simulink model "Ralenti_BO_End"  (R2024b)
settings: Solver=FixedStepAuto  StartTime=0.0  StopTime=80  FixedStep=10e-3  RelTol=1e-5  AbsTol=1e-6
values from neighbouring files (symbols this model uses):
  Copti = [0.4 1.0 1.5 2.9 3.5 4.1 5.2 5.4 7.5  8.5  9.1  9.9 10.1 11.8 11.9 ... (first row only)    [InitISM_AII.m]
  gam = 1.4    [InitISM_AII.m]
  J = 0.18    [InitISM_AII.m]
  Kv = 0.0016    [InitISM_AII.m]
  MAPtc = 0.03    [InitISM_AII.m]
  Mim0 = 0+0.001    (= 0.001)    [InitISM_AII.m]
  nv_remp = [0.090 0.110 0.120 0.110 0.130 0.150 0.135 0.155 0.140 0.145 0.140 0.135 0.120 0.120 ... (first row only)    [InitISM_AII.m]
  Pamb = 101300    [InitISM_AII.m]
  Pim0 = 0.8e5    (= 80000)    [InitISM_AII.m]
  PRcrit = ((gam+1)/2)^(gam/(1-gam))    (= 0.528281787717)    [InitISM_AII.m]
  Psens0 = 1e5    (= 100000)    [InitISM_AII.m]
  Rair = 287.0    (= 287)    [InitISM_AII.m]
  table_rdt_AA = [1.0000 0.9980 0.9955 0.9680 0.9500 0.9020 0.8195 0.6875 0.6080 0.5195 0.2000 0.0755]    [InitISM_AII.m]
  Tamb = 300    [InitISM_AII.m]
  Vcol = 0.0035    [InitISM_AII.m]
  Vcyl = 1998e-6/4    (= 0.0004995)    [InitISM_AII.m]
  vect_delta_AA = [0 2 3 8 10 14 19 25 28 31 40 43]    [InitISM_AII.m]
undefined symbols (not defined in the file or in its folder): N0
settings Model: Creator=a030141  LastModifiedBy=ramse
settings SolverCC: AutoScaleAbsTol=off  AlgebraicLoopSolver=TrustRegion
settings DataIOCC: SaveFormat=Array  SignalLoggingSaveFormat=ModelDataLogs  ReturnWorkspaceOutputs=off  SignalLoggingName=sigsOut
settings OptimizationCC: BlockReduction=off  BooleanDataType=off  ReuseModelBlockBuffer=off  ExpressionDepthLimit=2147483647  InitFltsAndDblsToZero=on  LifeSpan=inf
settings DebuggingCC: SaveWithParameterizedLinksMsg=none  UnderspecifiedInitializationDetection=Classic  MergeDetectMultiDrivingBlocksExec=none  SignalResolutionControl=TryResolveAllWithWarning  MultiTaskDSMMsg=warning  MultiTaskCondExecSysMsg=none  FcnCallInpInsideContextMsg=warning  UnconnectedInputMsg=warning  UnconnectedOutputMsg=warning  UnconnectedLineMsg=warning  StateNameClashWarn=warning  SFUnexpectedBacktrackingDiag=warning  SFNoUnconditionalDefaultTransitionDiag=warning  SFExecutionAtInitializationDiag=none  ArithmeticOperatorsInVariantConditions=warning
settings HardwareCC: ProdBitPerPointer=32  ProdBitPerSizeT=32  ProdBitPerPtrDiffT=32  ProdLargestAtomicFloat=None  ProdIntDivRoundTo=Undefined  ProdEndianess=Unspecified  ProdWordSize=32  ProdHWDeviceType=32-bit Generic  TargetUnknown=on
settings ModelReferenceCC: EnableRefExpFcnMdlSchedulingChecks=on  PropagateSignalLabelsOutOfModel=off
settings SFSimCC: SimUseLocalCustomCode=off  CustomCodeUndefinedFunction=UseInterfaceOnly
settings RTWCC: TemplateMakefile=grt_vc.tmf  RTWUseLocalCustomCode=off  GPUComputeCapability=3.5  DLArmComputeVersion=19.05
settings CodeAppCC: StateflowObjectComments=on
settings GRTTargetCC: TargetFcnLib=ansi_tfl_tmw.mat  TargetLangStandard=C89/C90 (ANSI)  CombineOutputUpdateFcns=off  GRTInterface=on
settings ConfigComp: CovMetricSettings=dw  CovSaveCumulativeToWorkspaceVar=on  CovSaveSingleToWorkspaceVar=on  CovExternalEMLEnable=off

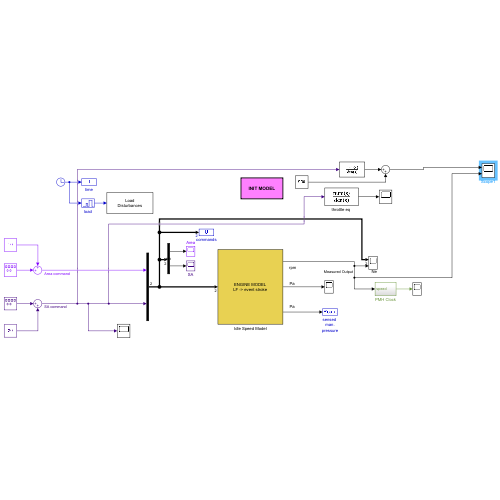
[thumbnail: Simulink's stored preview of the top-level diagram]
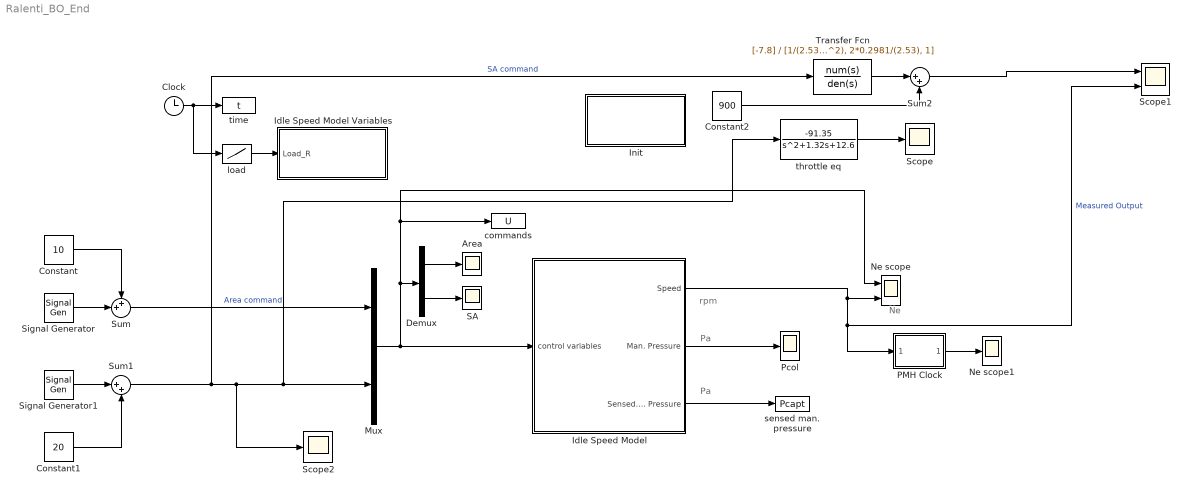
== system Ralenti_BO_End ==
  note: Pa
  note: Pa
  note: rpm
  note: Ne
  Area : Scope
  Clock : Clock
  Constant : Constant  Value=10  SampleTime=-1
  Constant1 : Constant  Value=20
  Constant2 : Constant  Value=900
  Demux : Demux  Outputs=2
      settings: DisplayOption=none
  Idle Speed Model : Subsystem
      mask Display: disp('ENGINE MODEL\nLF -> event stroke')
  Idle Speed Model Variables : Subsystem
      mask Display: disp('Load\nDisturbances')
  Init : Subsystem  TreatAsAtomicUnit=on
      settings: OpenFcn=InitISM_AII
      mask Display: disp('INIT MODEL')
  Mux : Mux  Inputs=2
  Ne scope : Scope  NumInputPorts=2
  Ne scope1 : Scope
  PMH Clock : Subsystem
  Pcol : Scope
  SA : Scope
  Scope : Scope
  Scope1 : Scope  NumInputPorts=2
  Scope2 : Scope
  Signal Generator : SignalGenerator  WaveForm=square  Amplitude=0  Frequency=0.01
  Signal Generator1 : SignalGenerator  WaveForm=square  Amplitude=2  Frequency=0.01
  Sum : Sum  Inputs=++|  SaturateOnIntegerOverflow=on
  Sum1 : Sum  Inputs=|++  SaturateOnIntegerOverflow=on
  Sum2 : Sum  Inputs=|++
  Transfer Fcn : TransferFcn  Numerator=[-7.8]  Denominator=[1/(2.53^2), 2*0.2981/(2.53), 1]
  commands : ToWorkspace  VariableName=U  SampleTime=-1
  load : Lookup  InputValues="[0  20 20 30 30 40 40 60 60 70]"  Table=[0 0 5 5 0 0 10 10 0 0]
  sensed man. pressure : ToWorkspace  VariableName=Pcapt  SampleTime=-1
  "throttle eq " : TransferFcn  Numerator=[-91.35]  Denominator=[1 1.32 12.6]
  time : ToWorkspace  VariableName=t  SampleTime=-1
  wires:
  Idle Speed Model/2(Man. Pressure) -> Pcol/1
  PMH Clock/1(out_1) -> Ne scope1/1
  Clock/1 -> time/1, load/1
  Idle Speed Model/3(Sensed Man. Pressure) -> sensed man. pressure/1
  Demux/1 -> Area/1
  Demux/2 -> SA/1
  load/1 -> Idle Speed Model Variables/1(Load_R)
  Mux/1 -> Idle Speed Model/1(control variables), Demux/1, Ne scope/1, commands/1
  Signal Generator1/1 -> Sum1/1
  Constant/1 -> Sum/1
  Constant1/1 -> Sum1/2
  Sum1/1 -> Transfer Fcn/1, Scope2/1, "throttle eq "/1, Mux/2  "SA command"
  Idle Speed Model/1(Speed) -> Ne scope/2, PMH Clock/1(speed), Scope1/2  "Measured Output"
  Sum/1 -> Mux/1  "Area command"
  Signal Generator/1 -> Sum/2
  "throttle eq "/1 -> Scope/1
  Transfer Fcn/1 -> Sum2/1
  Constant2/1 -> Sum2/2
  Sum2/1 -> Scope1/1

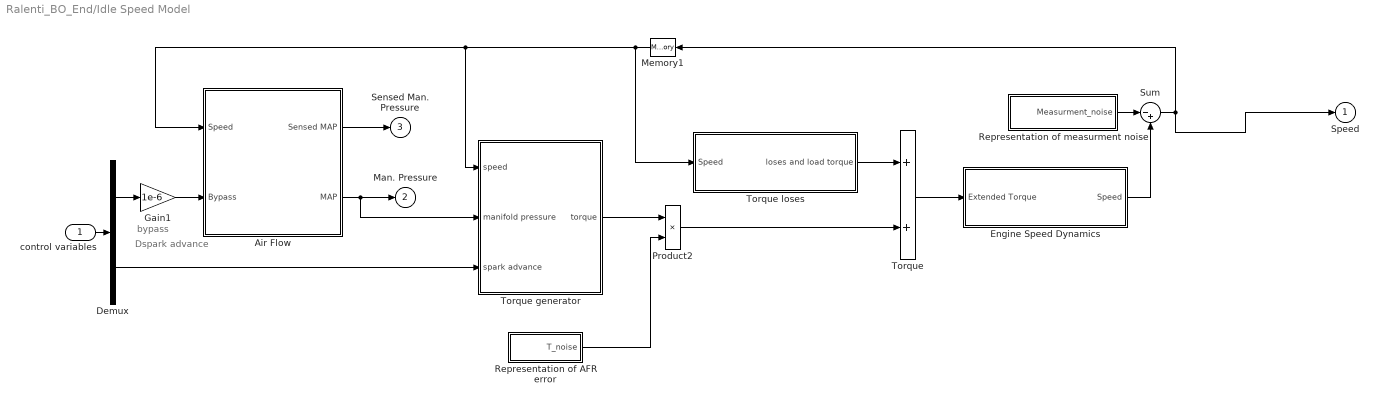
== system Ralenti_BO_End/Idle Speed Model ==
  note: Dspark advance
  note: bypass
  control variables : Inport
  " Torque loses" : Subsystem
  Air Flow : Subsystem
  Demux : Demux  Outputs=2
      settings: DisplayOption=none
  Engine Speed Dynamics : Subsystem
  Gain1 : Gain  Gain=1e-6  SaturateOnIntegerOverflow=on  OutDataTypeStr=Inherit: Same as input  ParamDataTypeStr=Inherit: Same as input
  Memory1 : Memory  InheritSampleTime=on
  Product2 : Product  Inputs=**  InputSameDT=on  SaturateOnIntegerOverflow=on  OutDataTypeStr=Inherit: Same as first input
  Representation of AFR error : Subsystem
  Representation of measurment noise : Subsystem
  Sum : Sum  Inputs=|-+  InputSameDT=on  SaturateOnIntegerOverflow=on  OutDataTypeStr=Inherit: Same as first input
  Torque : Sum  InputSameDT=on  SaturateOnIntegerOverflow=on  OutDataTypeStr=Inherit: Same as first input
  Torque generator : Subsystem
  Speed : Outport  VectorParamsAs1DForOutWhenUnconnected=off
  Man. Pressure : Outport  Port=2  VectorParamsAs1DForOutWhenUnconnected=off
  Sensed Man. Pressure : Outport  Port=3  VectorParamsAs1DForOutWhenUnconnected=off
  wires:
  Gain1/1 -> Air Flow/2(Bypass)
  Demux/1 -> Gain1/1
  Air Flow/2(MAP) -> Man. Pressure/1, Torque generator/2(manifold pressure)
  Air Flow/1(Sensed MAP) -> Sensed Man. Pressure/1
  Demux/2 -> Torque generator/3(spark advance)
  control variables/1 -> Demux/1
  Torque generator/1(torque) -> Product2/1
  Product2/1 -> Torque/2
  Representation of AFR error/1(T_noise) -> Product2/2
  Representation of measurment noise/1(Measurment_noise) -> Sum/1
  " Torque loses"/1(loses and load torque) -> Torque/1
  Torque/1 -> Engine Speed Dynamics/1(Extended Torque)
  Engine Speed Dynamics/1(Speed) -> Sum/2
  Memory1/1 -> Air Flow/1(Speed), Torque generator/1(speed), " Torque loses"/1(Speed)
  Sum/1 -> Speed/1, Memory1/1

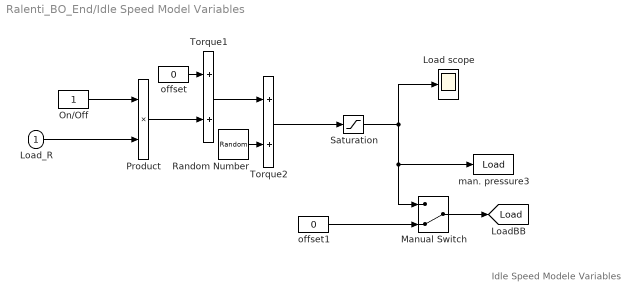
== system Ralenti_BO_End/Idle Speed Model Variables ==
  note: Idle Speed Modele Variables
  Load_R : Inport
  Load scope : Scope
  Manual Switch : ManualSwitch  CurrentSetting=0
  On/Off : Constant
  Product : Product  InputSameDT=on  SaturateOnIntegerOverflow=on  OutDataTypeStr=Inherit: Same as first input
  Random Number : RandomNumber  Variance=0.001  SampleTime=0.01
  Saturation : Saturate  UpperLimit=30  LowerLimit=0
  Torque1 : Sum  InputSameDT=on  SaturateOnIntegerOverflow=on  OutDataTypeStr=Inherit: Same as first input
  Torque2 : Sum  InputSameDT=on  SaturateOnIntegerOverflow=on  OutDataTypeStr=Inherit: Same as first input
  man. pressure3 : ToWorkspace  VariableName=Load  SampleTime=-1
  offset : Constant  Value=0
  offset1 : Constant  Value=0
  tag scope: Load=global
  wires:
  On/Off/1 -> Product/1
  Load_R/1 -> Product/2
  Product/1 -> Torque1/2
  offset/1 -> Torque1/1
  Random Number/1 -> Torque2/2
  Torque1/1 -> Torque2/1
  Saturation/1 -> Load scope/1, man. pressure3/1, Manual Switch/1
  Torque2/1 -> Saturation/1
  Manual Switch/1 -> [Load]
  offset1/1 -> Manual Switch/2

== system Ralenti_BO_End/Init ==

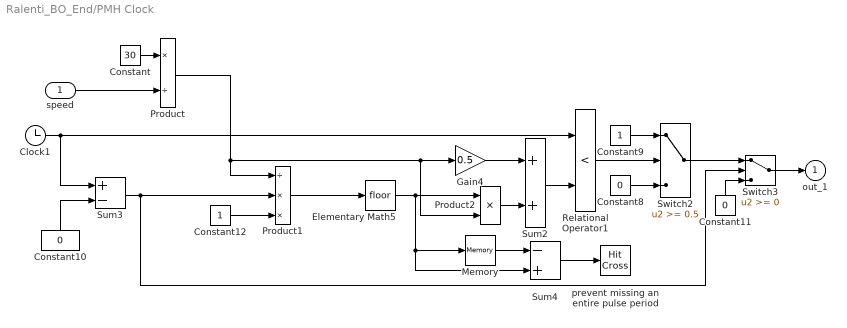
== system Ralenti_BO_End/PMH Clock ==
  speed : Inport
  Clock1 : Clock
  Constant : Constant  Value=30
  Constant10 : Constant  Value=0
  Constant11 : Constant  Value=0
  Constant12 : Constant
  Constant8 : Constant  Value=0
  Constant9 : Constant
  Elementary Math5 : Rounding
  Gain4 : Gain  Gain=0.5  SaturateOnIntegerOverflow=on  OutDataTypeStr=Inherit: Same as input  ParamDataTypeStr=Inherit: Same as input
  Memory : Memory
  Product : Product  Inputs=*/  InputSameDT=on  SaturateOnIntegerOverflow=on  OutDataTypeStr=Inherit: Same as first input
  Product1 : Product  Inputs=/**  InputSameDT=on  SaturateOnIntegerOverflow=on  OutDataTypeStr=Inherit: Same as first input
  Product2 : Product  InputSameDT=on  SaturateOnIntegerOverflow=on  OutDataTypeStr=Inherit: Same as first input
  Relational Operator1 : RelationalOperator  Operator=<
  Sum2 : Sum  InputSameDT=on  SaturateOnIntegerOverflow=on  OutDataTypeStr=Inherit: Same as first input
  Sum3 : Sum  Inputs=+-  InputSameDT=on  SaturateOnIntegerOverflow=on  OutDataTypeStr=Inherit: Same as first input
  Sum4 : Sum  Inputs=-+  InputSameDT=on  SaturateOnIntegerOverflow=on  OutDataTypeStr=Inherit: Same as first input
  Switch2 : Switch  Threshold=0.5
  Switch3 : Switch
  prevent missing an entire pulse period : HitCross  HitCrossingOffset=1  ShowOutputPort=off
  out_1 : Outport  VectorParamsAs1DForOutWhenUnconnected=off
  wires:
  Elementary Math5/1 -> Sum4/2, Memory/1, Product2/1
  Gain4/1 -> Sum2/1
  Product1/1 -> Elementary Math5/1
  Switch2/1 -> Switch3/1
  Constant11/1 -> Switch3/3
  Constant9/1 -> Switch2/1
  Constant8/1 -> Switch2/3
  Relational Operator1/1 -> Switch2/2
  Switch3/1 -> out_1/1
  Sum2/1 -> Relational Operator1/2
  Clock1/1 -> Relational Operator1/1, Sum3/1
  Sum3/1 -> Switch3/2, Product1/2
  Constant10/1 -> Sum3/2
  Memory/1 -> Sum4/1
  Sum4/1 -> prevent missing an entire pulse period/1
  Product2/1 -> Sum2/2
  Constant12/1 -> Product1/3
  Constant/1 -> Product/1
  speed/1 -> Product/2
  Product/1 -> Product1/1, Gain4/1, Product2/2

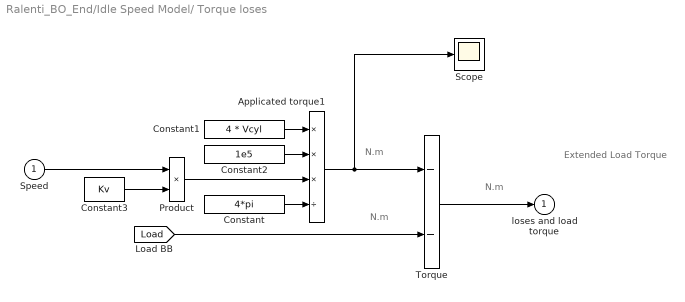
== system Ralenti_BO_End/Idle Speed Model/ Torque loses ==
  note: N.m
  note: Extended Load Torque
  note: N.m
  note: N.m
  Speed : Inport
  Applicated torque1 : Product  Inputs=***/  InputSameDT=on  SaturateOnIntegerOverflow=on  OutDataTypeStr=Inherit: Same as first input
  Constant : Constant  Value=4*pi
  Constant1 : Constant  Value=4 * Vcyl
  Constant2 : Constant  Value=1e5
  Constant3 : Constant  Value=Kv
  Product : Product  Inputs=**  InputSameDT=on  RndMeth=Zero  SaturateOnIntegerOverflow=on  OutDataTypeStr=Inherit: Same as first input
  Scope : Scope
  Torque : Sum  Inputs=--  InputSameDT=on  SaturateOnIntegerOverflow=on  OutDataTypeStr=Inherit: Same as first input
  loses and load torque : Outport  VectorParamsAs1DForOutWhenUnconnected=off
  wires:
  Constant3/1 -> Product/2
  Speed/1 -> Product/1
  [Load] -> Torque/2
  Torque/1 -> loses and load torque/1
  Product/1 -> Applicated torque1/3
  Applicated torque1/1 -> Torque/1, Scope/1
  Constant/1 -> Applicated torque1/4
  Constant1/1 -> Applicated torque1/1
  Constant2/1 -> Applicated torque1/2

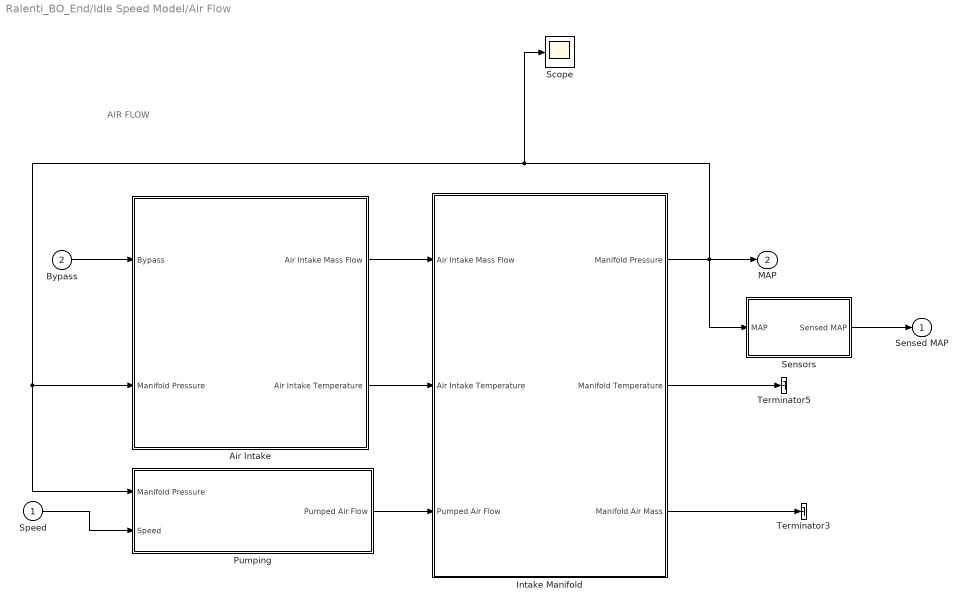
== system Ralenti_BO_End/Idle Speed Model/Air Flow ==
  note: AIR FLOW
  Speed : Inport
  Bypass : Inport  Port=2
  Air Intake : Subsystem
  Intake Manifold : Subsystem
  Pumping : Subsystem
  Scope : Scope
  Sensors : Subsystem
  Terminator3 : Terminator
  Terminator5 : Terminator
  Sensed MAP : Outport  VectorParamsAs1DForOutWhenUnconnected=off
  MAP : Outport  Port=2  VectorParamsAs1DForOutWhenUnconnected=off
  wires:
  Pumping/1(Pumped Air Flow) -> Intake Manifold/3(Pumped Air Flow)
  Sensors/1(Sensed MAP) -> Sensed MAP/1
  Air Intake/1(Air Intake Mass Flow) -> Intake Manifold/1(Air Intake Mass Flow)
  Bypass/1 -> Air Intake/1(Bypass)
  Air Intake/2(Air Intake Temperature) -> Intake Manifold/2(Air Intake Temperature)
  Intake Manifold/2(Manifold Temperature) -> Terminator5/1
  Intake Manifold/3(Manifold Air Mass) -> Terminator3/1
  Speed/1 -> Pumping/2(Speed)
  Intake Manifold/1(Manifold Pressure) -> MAP/1, Sensors/1(MAP), Scope/1, Pumping/1(Manifold Pressure), Air Intake/2(Manifold Pressure)

== system Ralenti_BO_End/Idle Speed Model/Engine Speed Dynamics ==
  note: Engine Speed
  note: Tr/min
  note: rad/s
  Extended Torque : Inport
  Constant : Constant  Value=J
  Product1 : Product  Inputs=*/  InputSameDT=on  SaturateOnIntegerOverflow=on  OutDataTypeStr=Inherit: Same as first input
  integrator : Integrator  InitialCondition=N0  UpperSaturationLimit=100  LowerSaturationLimit=0
  speed unit conversion : Gain  Gain=30/pi  SaturateOnIntegerOverflow=on  OutDataTypeStr=Inherit: Same as input  ParamDataTypeStr=Inherit: Same as input
  Speed : Outport  VectorParamsAs1DForOutWhenUnconnected=off
  wires:
  Constant/1 -> Product1/2
  Extended Torque/1 -> Product1/1
  Product1/1 -> speed unit conversion/1
  speed unit conversion/1 -> integrator/1
  integrator/1 -> Speed/1

== system Ralenti_BO_End/Idle Speed Model/Representation of AFR error ==
  Constant : Constant
  Random Number : RandomNumber  Variance=0  SampleTime=0.01
  Sum : Sum  Inputs=|-+  InputSameDT=on  SaturateOnIntegerOverflow=on  OutDataTypeStr=Inherit: Same as first input
  T_noise : Outport  VectorParamsAs1DForOutWhenUnconnected=off
  wires:
  Random Number/1 -> Sum/1
  Sum/1 -> T_noise/1
  Constant/1 -> Sum/2

== system Ralenti_BO_End/Idle Speed Model/Representation of measurment noise ==
  Random Number : RandomNumber  Variance=0.1
  gain _noise : Gain  Gain=0  SaturateOnIntegerOverflow=on  OutDataTypeStr=Inherit: Same as input
  Measurment_noise : Outport  VectorParamsAs1DForOutWhenUnconnected=off
  wires:
  Random Number/1 -> gain _noise/1
  gain _noise/1 -> Measurment_noise/1

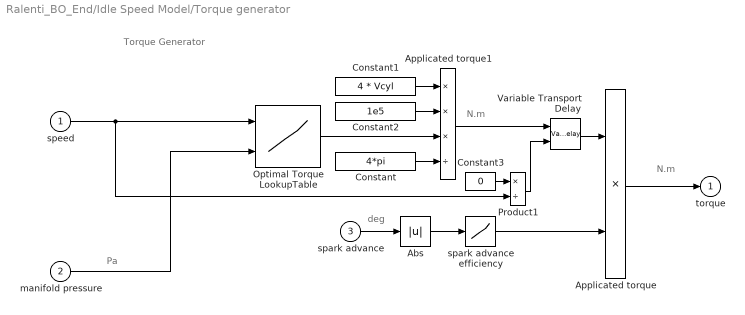
== system Ralenti_BO_End/Idle Speed Model/Torque generator ==
  note: Torque Generator
  note: N.m
  note: N.m
  note: deg
  note: Pa
  speed : Inport
  manifold pressure : Inport  Port=2
  spark advance : Inport  Port=3
  Abs : Abs
  Applicated torque : Product  InputSameDT=on  SaturateOnIntegerOverflow=on  OutDataTypeStr=Inherit: Same as first input
  Applicated torque1 : Product  Inputs=***/  InputSameDT=on  SaturateOnIntegerOverflow=on  OutDataTypeStr=Inherit: Same as first input
  Constant : Constant  Value=4*pi
  Constant1 : Constant  Value=4 * Vcyl
  Constant2 : Constant  Value=1e5
  Constant3 : Constant  Value=0
  Optimal Torque LookupTable : Lookup2D  RowIndex=Ne_remp  ColumnIndex=Pcol_remp  Table=Copti
  Product1 : Product  Inputs=*/  SaturateOnIntegerOverflow=on  OutDataTypeStr=Inherit: Same as first input
  Variable Transport Delay : VariableTransportDelay  MaximumDelay=10  InitialOutput=10
  spark advance efficiency : Lookup  InputValues=vect_delta_AA  Table=table_rdt_AA
  torque : Outport  VectorParamsAs1DForOutWhenUnconnected=off
  wires:
  spark advance/1 -> Abs/1
  Applicated torque/1 -> torque/1
  speed/1 -> Optimal Torque LookupTable/1, Product1/2
  Abs/1 -> spark advance efficiency/1
  manifold pressure/1 -> Optimal Torque LookupTable/2
  spark advance efficiency/1 -> Applicated torque/2
  Optimal Torque LookupTable/1 -> Applicated torque1/3
  Constant/1 -> Applicated torque1/4
  Constant1/1 -> Applicated torque1/1
  Constant2/1 -> Applicated torque1/2
  Applicated torque1/1 -> Variable Transport Delay/1
  Variable Transport Delay/1 -> Applicated torque/1
  Constant3/1 -> Product1/1
  Product1/1 -> Variable Transport Delay/2

== system Ralenti_BO_End/Idle Speed Model/Air Flow/Air Intake ==
  note: AIR INTAKE
  note: m^2
  note: kg/s
  note: Pa
  note: K
  Bypass : Inport
  Manifold Pressure : Inport  Port=2
  Compressible Flow Equation : Subsystem
  Product : Product  InputSameDT=on  SaturateOnIntegerOverflow=on  OutDataTypeStr=Inherit: Same as first input
  Air Intake Mass Flow : Outport  VectorParamsAs1DForOutWhenUnconnected=off
  Air Intake Temperature : Outport  Port=2  VectorParamsAs1DForOutWhenUnconnected=off
  wires:
  Product/1 -> Air Intake Mass Flow/1
  Manifold Pressure/1 -> Compressible Flow Equation/1(Manifold Pressure)
  Compressible Flow Equation/1(Air Intake Mass Flow) -> Product/2
  Bypass/1 -> Product/1
  Compressible Flow Equation/2(Air Intake Temperature) -> Air Intake Temperature/1

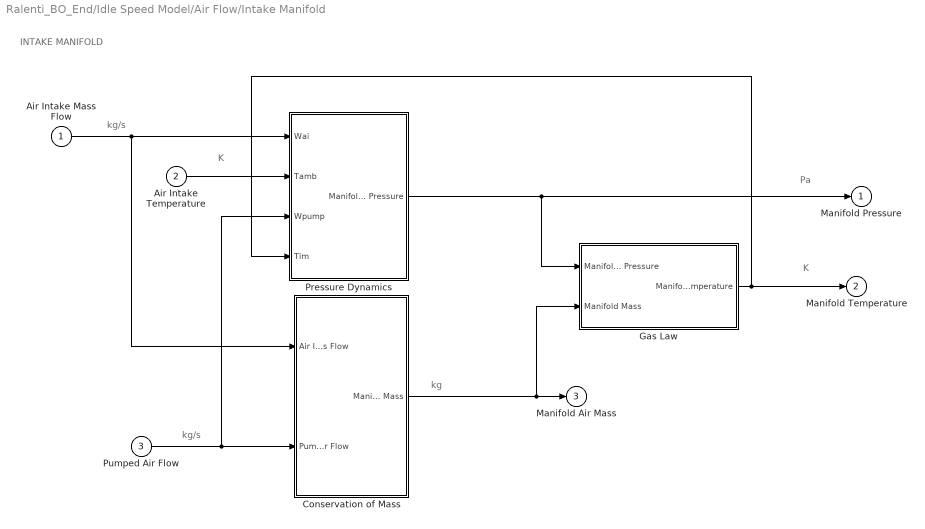
== system Ralenti_BO_End/Idle Speed Model/Air Flow/Intake Manifold ==
  note: INTAKE MANIFOLD
  note: kg/s
  note: K
  note: kg/s
  note: kg
  note: Pa
  note: K
  Air Intake Mass Flow : Inport
  Air Intake Temperature : Inport  Port=2
  Pumped Air Flow : Inport  Port=3
  Conservation of Mass : Subsystem
  Gas Law : Subsystem
  Pressure Dynamics : Subsystem
  Manifold Pressure : Outport  VectorParamsAs1DForOutWhenUnconnected=off
  Manifold Temperature : Outport  Port=2  VectorParamsAs1DForOutWhenUnconnected=off
  Manifold Air Mass : Outport  Port=3  VectorParamsAs1DForOutWhenUnconnected=off
  wires:
  Gas Law/1(Manifold Temperature) -> Manifold Temperature/1, Pressure Dynamics/4(Tim)
  Pumped Air Flow/1 -> Pressure Dynamics/3(Wpump), Conservation of Mass/2(Pumped Air Flow)
  Air Intake Temperature/1 -> Pressure Dynamics/2(Tamb)
  Pressure Dynamics/1(Manifold Pressure) -> Manifold Pressure/1, Gas Law/1(Manifold Pressure)
  Air Intake Mass Flow/1 -> Pressure Dynamics/1(Wai), Conservation of Mass/1(Air Intake Mass Flow)
  Conservation of Mass/1(Manifold Mass) -> Manifold Air Mass/1, Gas Law/2("Manifold Mass ")

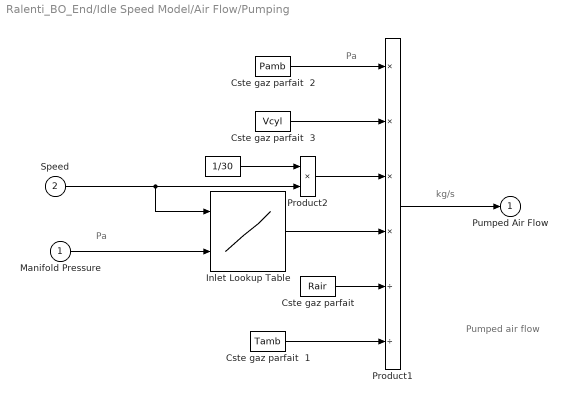
== system Ralenti_BO_End/Idle Speed Model/Air Flow/Pumping ==
  note: Pumped air flow
  note: kg/s
  note: Pa
  note: Pa
  Manifold Pressure : Inport
  Speed : Inport  Port=2
  " " : Constant  Value=1/30
  "Cste gaz parfait  " : Constant  Value=Rair
  Cste gaz parfait  1 : Constant  Value=Tamb
  Cste gaz parfait  2 : Constant  Value=Pamb
  Cste gaz parfait  3 : Constant  Value=Vcyl
  Inlet Lookup Table : Lookup2D  RowIndex=Ne_remp  ColumnIndex=Pcol_remp  Table=nv_remp
  Product1 : Product  Inputs=****//  InputSameDT=on  SaturateOnIntegerOverflow=on  OutDataTypeStr=Inherit: Same as first input
  Product2 : Product  InputSameDT=on  SaturateOnIntegerOverflow=on  OutDataTypeStr=Inherit: Same as first input
  Pumped Air Flow : Outport  VectorParamsAs1DForOutWhenUnconnected=off
  wires:
  Product1/1 -> Pumped Air Flow/1
  " "/1 -> Product2/1
  Speed/1 -> Inlet Lookup Table/1, Product2/2
  Inlet Lookup Table/1 -> Product1/4
  Cste gaz parfait  3/1 -> Product1/2
  Product2/1 -> Product1/3
  "Cste gaz parfait  "/1 -> Product1/5
  Manifold Pressure/1 -> Inlet Lookup Table/2
  Cste gaz parfait  1/1 -> Product1/6
  Cste gaz parfait  2/1 -> Product1/1

== system Ralenti_BO_End/Idle Speed Model/Air Flow/Sensors ==
  note: SENSORS
  MAP : Inport
  Gain1 : Gain  Gain=1/MAPtc  SaturateOnIntegerOverflow=on  OutDataTypeStr=Inherit: Same as input  ParamDataTypeStr=Inherit: Same as input
  Integrator1 : Integrator  InitialCondition=Psens0
  Sum1 : Sum  Inputs=-+  InputSameDT=on  SaturateOnIntegerOverflow=on  OutDataTypeStr=Inherit: Same as first input
  Sensed MAP : Outport  VectorParamsAs1DForOutWhenUnconnected=off
  wires:
  MAP/1 -> Sum1/2
  Gain1/1 -> Integrator1/1
  Sum1/1 -> Gain1/1
  Integrator1/1 -> Sensed MAP/1, Sum1/1

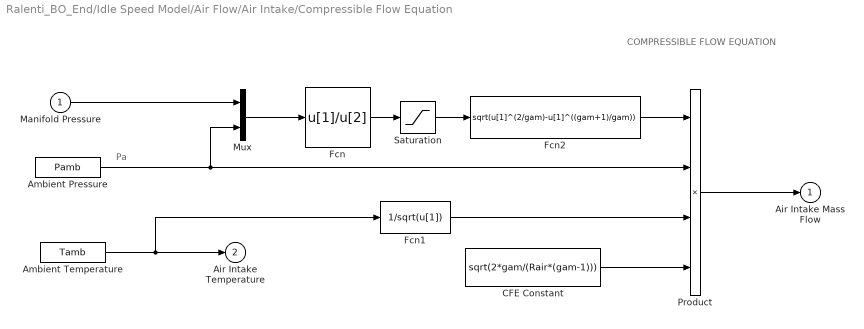
== system Ralenti_BO_End/Idle Speed Model/Air Flow/Air Intake/Compressible Flow Equation ==
  note: COMPRESSIBLE FLOW EQUATION
  note: Pa
  Manifold Pressure : Inport
  Ambient Pressure : Constant  Value=Pamb
  Ambient Temperature : Constant  Value=Tamb
  "CFE Constant " : Constant  Value=sqrt(2*gam/(Rair*(gam-1)))
  Fcn : Fcn  Expr=u[1]/u[2]
  Fcn1 : Fcn  Expr=1/sqrt(u[1])
  Fcn2 : Fcn  Expr=sqrt(u[1]^(2/gam)-u[1]^((gam+1)/gam))
  Mux : Mux  Inputs=2
  Product : Product  Inputs=4  InputSameDT=on  SaturateOnIntegerOverflow=on  OutDataTypeStr=Inherit: Same as first input
  Saturation : Saturate  UpperLimit=1  LowerLimit=PRcrit
  Air Intake Mass Flow : Outport  VectorParamsAs1DForOutWhenUnconnected=off
  Air Intake Temperature : Outport  Port=2  VectorParamsAs1DForOutWhenUnconnected=off
  wires:
  Ambient Pressure/1 -> Product/2, Mux/2
  Product/1 -> Air Intake Mass Flow/1
  "CFE Constant "/1 -> Product/4
  Fcn2/1 -> Product/1
  Saturation/1 -> Fcn2/1
  Fcn1/1 -> Product/3
  Fcn/1 -> Saturation/1
  Mux/1 -> Fcn/1
  Manifold Pressure/1 -> Mux/1
  Ambient Temperature/1 -> Fcn1/1, Air Intake Temperature/1

== system Ralenti_BO_End/Idle Speed Model/Air Flow/Intake Manifold/Conservation of Mass ==
  note: CONVERSION OF MASS
  Air Intake Mass Flow : Inport
  Pumped Air Flow : Inport  Port=2
  Integrator : Integrator  InitialCondition=Mim0
  Sum : Sum  Inputs=+-  InputSameDT=on  SaturateOnIntegerOverflow=on  OutDataTypeStr=Inherit: Same as first input
  Manifold Mass : Outport  VectorParamsAs1DForOutWhenUnconnected=off
  wires:
  Integrator/1 -> Manifold Mass/1
  Sum/1 -> Integrator/1
  Pumped Air Flow/1 -> Sum/2
  Air Intake Mass Flow/1 -> Sum/1

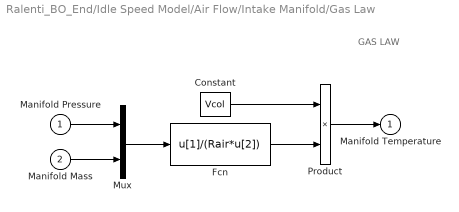
== system Ralenti_BO_End/Idle Speed Model/Air Flow/Intake Manifold/Gas Law ==
  note: GAS LAW
  Manifold Pressure : Inport
  "Manifold Mass " : Inport  Port=2
  Constant : Constant  Value=Vcol
  Fcn : Fcn  Expr=u[1]/(Rair*u[2])
  Mux : Mux  Inputs=2
  Product : Product  InputSameDT=on  SaturateOnIntegerOverflow=on  OutDataTypeStr=Inherit: Same as first input
  Manifold Temperature : Outport  VectorParamsAs1DForOutWhenUnconnected=off
  wires:
  Mux/1 -> Fcn/1
  Manifold Pressure/1 -> Mux/1
  Fcn/1 -> Product/2
  Product/1 -> Manifold Temperature/1
  Constant/1 -> Product/1
  "Manifold Mass "/1 -> Mux/2

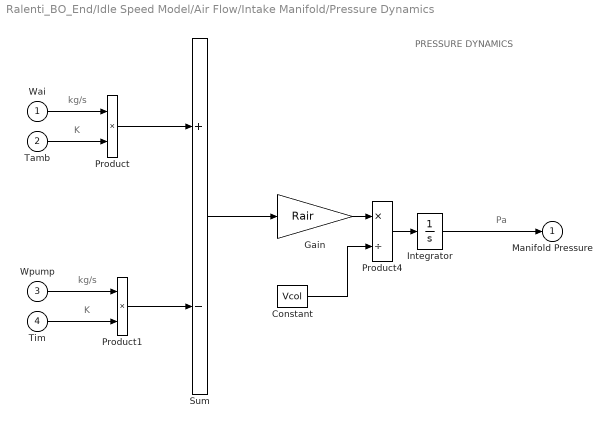
== system Ralenti_BO_End/Idle Speed Model/Air Flow/Intake Manifold/Pressure Dynamics ==
  note: PRESSURE DYNAMICS
  note: kg/s
  note: K
  note: kg/s
  note: K
  note: Pa
  Wai : Inport
  Tamb : Inport  Port=2
  Wpump : Inport  Port=3
  Tim : Inport  Port=4
  Constant : Constant  Value=Vcol
  Gain : Gain  Gain=Rair  SaturateOnIntegerOverflow=on  OutDataTypeStr=Inherit: Same as input  ParamDataTypeStr=Inherit: Same as input
  Integrator : Integrator  InitialCondition=Pim0
  Product : Product  InputSameDT=on  SaturateOnIntegerOverflow=on  OutDataTypeStr=Inherit: Same as first input
  Product1 : Product  InputSameDT=on  SaturateOnIntegerOverflow=on  OutDataTypeStr=Inherit: Same as first input
  Product4 : Product  Inputs=*/  InputSameDT=on  SaturateOnIntegerOverflow=on  OutDataTypeStr=Inherit: Same as first input
  Sum : Sum  Inputs=+-  InputSameDT=on  SaturateOnIntegerOverflow=on  OutDataTypeStr=Inherit: Same as first input
  Manifold Pressure : Outport  VectorParamsAs1DForOutWhenUnconnected=off
  wires:
  Sum/1 -> Gain/1
  Product1/1 -> Sum/2
  Product/1 -> Sum/1
  Tim/1 -> Product1/2
  Wpump/1 -> Product1/1
  Tamb/1 -> Product/2
  Wai/1 -> Product/1
  Gain/1 -> Product4/1
  Integrator/1 -> Manifold Pressure/1
  Product4/1 -> Integrator/1
  Constant/1 -> Product4/2
